simulink model "buck_PV_matematico"  (R2024a)
settings: Solver=FixedStepAuto  StartTime=0.0  StopTime=0.3  FixedStep=1/150000  RelTol=1e-3
values from neighbouring files (symbols this model uses):
  alpha = 0.003177    [parametros.m]
  Cin = 2.7e-3    (= 0.0027)    [parametros.m]
  EG = 1.12    [parametros.m]
  eta = 1.4    [parametros.m]
  Irr = 1.26e-8    (= 1.26e-08)    [parametros.m]
  Isc = 8.21    [parametros.m]
  k = 1.38E-23    (= 1.38e-23)    [parametros.m]
  kdE = 0.1    [parametros.m]
  kE = 0.3333    [parametros.m]
  ki = zeros(n_pontos,n_pontos)    [FLS_dados.m]
  ki_0 = 3.23    [parametros.m]
  kki = 1.5    [parametros.m]
  kkp = 0.0015    [parametros.m]
  kp = zeros(n_pontos,n_pontos)    [FLS_dados.m]
  kp_0 = 0.0055    [parametros.m]
  L = 22.109e-6    (= 2.2109e-05)    [parametros.m]
  n_cell = 45    [parametros.m]
  n_pontos = 21    [FLS_dados.m]
  q = 1.6E-19    (= 1.6e-19)    [parametros.m]
  Rcin = 6.519e-3    (= 0.006519)    [parametros.m]
  Rl = 3e-3    (= 0.003)    [parametros.m]
  Ron = 0.15    [parametros.m]
  Rp_cell = 2.116    [parametros.m]
  Rs_cell = 0.0045    [parametros.m]
  Tr = 298    [parametros.m]
  Vbat = 12    [parametros.m]
  Vto = 1    [parametros.m]
libraries: simulink x1
settings Model: Creator=mario  LastModifiedBy=mario

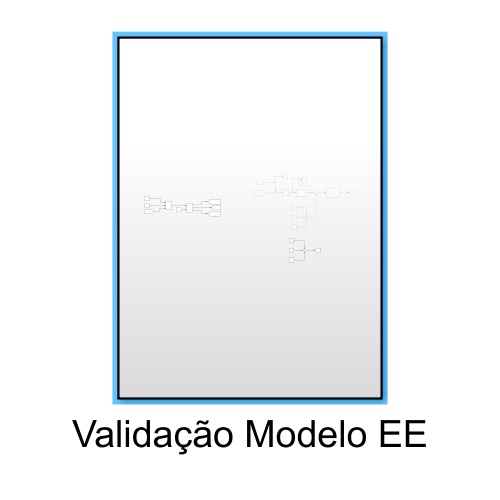
[thumbnail: Simulink's stored preview of the top-level diagram]
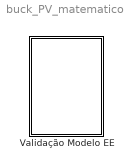
== system buck_PV_matematico ==
  Validação Modelo EE : Subsystem

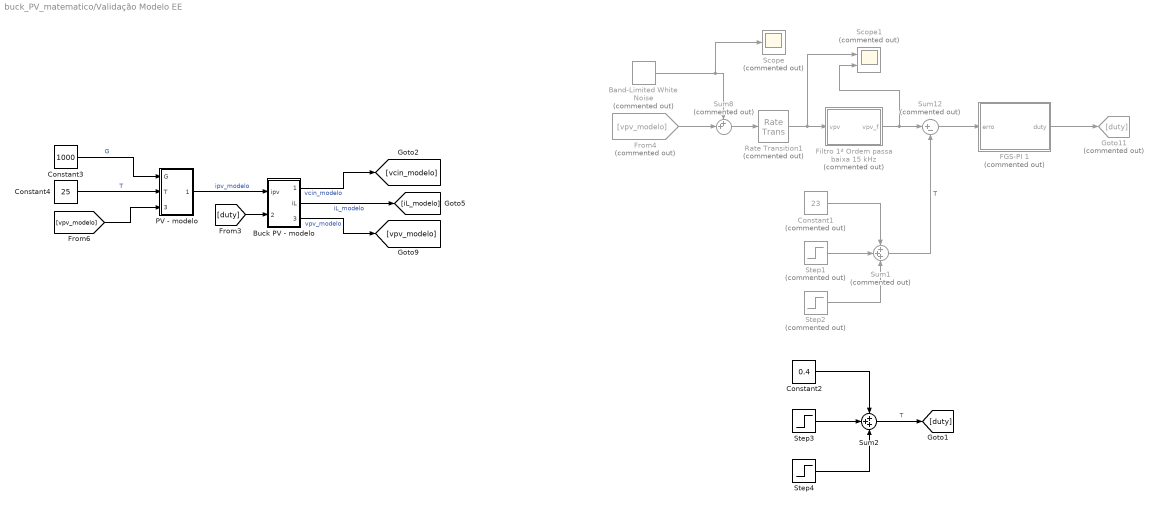
== system buck_PV_matematico/Validação Modelo EE ==
  Band-Limited White Noise : simulink/Sources/Band-Limited White Noise  Commented=on  Cov=[5e-7]  Ts=(1/150000)  seed=[23341]
  Buck PV - modelo : Subsystem
  Constant1 : Constant  Commented=on  Value=23
  Constant2 : Constant  Value=0.4
  Constant3 : Constant  Value=1000
  Constant4 : Constant  Value=25
  FGS-PI 1 : Subsystem  Commented=on
  Filtro 1ª Ordem passa baixa 15 kHz : MATLAB Function  Commented=on  TreatAsAtomicUnit=on
  From4 : From  Commented=on  GotoTag=vpv_modelo
  Goto11 : Goto  Commented=on  GotoTag=duty
  PV - modelo : Subsystem
  Rate Transition1 : RateTransition  Commented=on  OutPortSampleTime=1/150000
  Scope : Scope  Commented=on
  Scope1 : Scope  Commented=on  NumInputPorts=2
  Step1 : Step  Commented=on  Time=0.1  After=3  SampleTime=0
  Step2 : Step  Commented=on  Time=0.2  After=-3  SampleTime=0
  Step3 : Step  Time=0.1  After=0.01  SampleTime=0
  Step4 : Step  Time=0.2  After=-0.01  SampleTime=0
  Sum1 : Sum  Commented=on  Inputs=+++
  Sum12 : Sum  Commented=on  Inputs=|+-
  Sum2 : Sum  Inputs=+++
  Sum8 : Sum  Commented=on  Inputs=++|
  wires:
  PV - modelo/1(Ipv) -> Buck PV - modelo/1(ipv)  "ipv_modelo"
  [duty] -> Buck PV - modelo/2(duty)
  Buck PV - modelo/1(vcin) -> [vcin_modelo]  "vcin_modelo"
  [vpv_modelo] -> PV - modelo/3(Vpv)
  Constant4/1 -> PV - modelo/2(T)  "T"
  Buck PV - modelo/2(iL) -> [iL_modelo]  "iL_modelo"
  Buck PV - modelo/3(vpv) -> [vpv_modelo]  "vpv_modelo"
  Constant3/1 -> PV - modelo/1(G)  "G"
  FGS-PI 1/1(duty) -> Goto11/1
  From4/1 -> Sum8/2
  Band-Limited White Noise/1 -> Scope/1, Sum8/1
  Rate Transition1/1 -> Scope1/1, Filtro 1ª Ordem passa baixa 15 kHz/1(vpv)
  Sum8/1 -> Rate Transition1/1
  Filtro 1ª Ordem passa baixa 15 kHz/1(vpv_f) -> Scope1/2, Sum12/1
  Sum12/1 -> FGS-PI 1/1(erro)
  Step1/1 -> Sum1/2
  Sum1/1 -> Sum12/2  "T"
  Constant1/1 -> Sum1/1
  Step2/1 -> Sum1/3
  Step4/1 -> Sum2/3
  Constant2/1 -> Sum2/1
  Step3/1 -> Sum2/2
  Sum2/1 -> [duty]  "T"

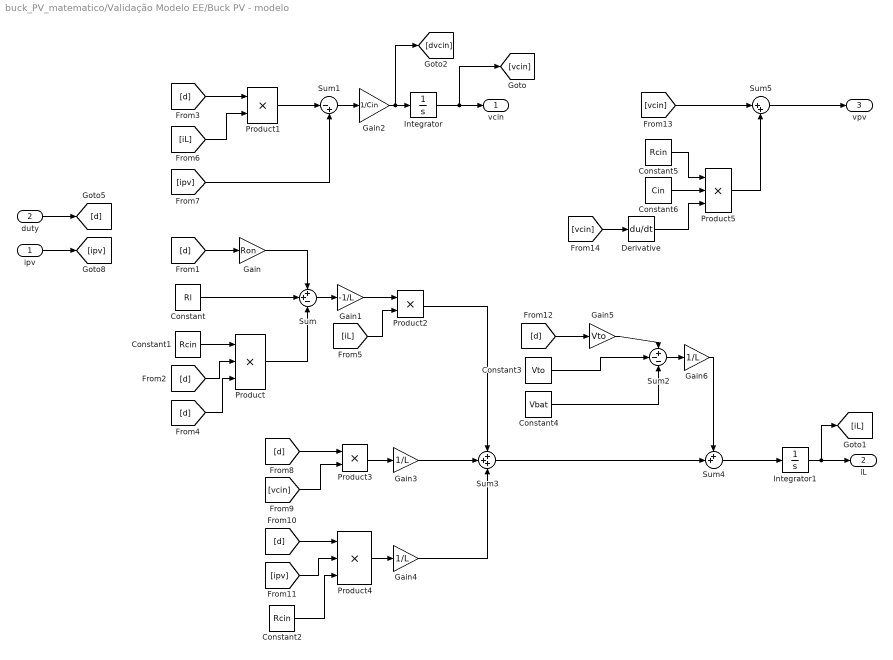
== system buck_PV_matematico/Validação Modelo EE/Buck PV - modelo ==
  ipv : Inport
  duty : Inport  Port=2
  Constant : Constant  Value=Rl
  Constant1 : Constant  Value=Rcin
  Constant2 : Constant  Value=Rcin
  Constant3 : Constant  Value=Vto
  Constant4 : Constant  Value=Vbat
  Constant5 : Constant  Value=Rcin
  Constant6 : Constant  Value=Cin
  Derivative : Derivative
  Gain : Gain  Gain=Ron
  Gain1 : Gain  Gain=-1/L
  Gain2 : Gain  Gain=1/Cin
  Gain3 : Gain  Gain=1/L
  Gain4 : Gain  Gain=1/L
  Gain5 : Gain  Gain=Vto
  Gain6 : Gain  Gain=1/L
  Integrator : Integrator
  Integrator1 : Integrator
  Product : Product  Inputs=3
  Product1 : Product
  Product2 : Product
  Product3 : Product
  Product4 : Product  Inputs=3
  Product5 : Product  Inputs=3
  Sum : Sum  Inputs=++-
  Sum1 : Sum  Inputs=|-+
  Sum2 : Sum  Inputs=+--
  Sum3 : Sum  Inputs=+++
  Sum4 : Sum  Inputs=++|
  Sum5 : Sum  Inputs=|++
  vcin : Outport
  iL : Outport  Port=2
  vpv : Outport  Port=3
  wires:
  ipv/1 -> [ipv]
  duty/1 -> [d]
  Integrator/1 -> [vcin], vcin/1
  Product1/1 -> Sum1/1
  Sum1/1 -> Gain2/1
  [d] -> Product1/1
  [iL] -> Product1/2
  [ipv] -> Sum1/2
  Gain2/1 -> [dvcin], Integrator/1
  [d] -> Gain/1
  Gain/1 -> Sum/1
  Constant/1 -> Sum/2
  Constant1/1 -> Product/1
  [d] -> Product/2
  [d] -> Product/3
  Product/1 -> Sum/3
  Sum/1 -> Gain1/1
  Gain1/1 -> Product2/1
  [iL] -> Product2/2
  [d] -> Product3/1
  [vcin] -> Product3/2
  Product3/1 -> Gain3/1
  [d] -> Product4/1
  [ipv] -> Product4/2
  Constant2/1 -> Product4/3
  Product4/1 -> Gain4/1
  [d] -> Gain5/1
  Gain5/1 -> Sum2/1
  Constant3/1 -> Sum2/2
  Constant4/1 -> Sum2/3
  Gain3/1 -> Sum3/2
  Gain4/1 -> Sum3/3
  Product2/1 -> Sum3/1
  Sum3/1 -> Sum4/2
  Sum2/1 -> Gain6/1
  Sum4/1 -> Integrator1/1
  Integrator1/1 -> [iL], iL/1
  Gain6/1 -> Sum4/1
  [vcin] -> Sum5/1
  Constant6/1 -> Product5/2
  Constant5/1 -> Product5/1
  [vcin] -> Derivative/1
  Product5/1 -> Sum5/2
  Sum5/1 -> vpv/1
  Derivative/1 -> Product5/3

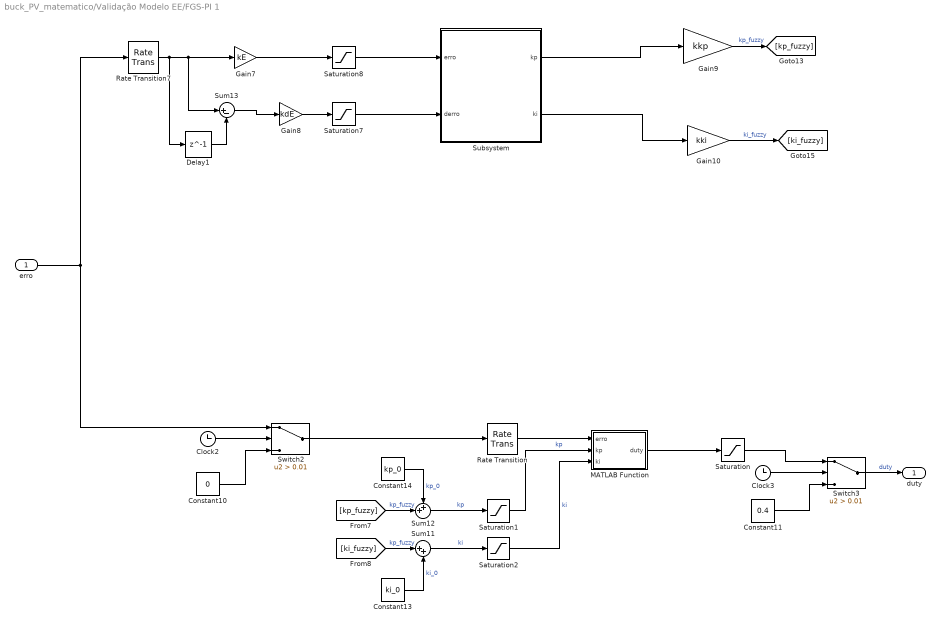
== system buck_PV_matematico/Validação Modelo EE/FGS-PI 1 ==
  erro : Inport
  Clock2 : Clock
  Clock3 : Clock
  Constant10 : Constant  Value=0
  Constant11 : Constant  Value=0.4
  Constant13 : Constant  Value=ki_0
  Constant14 : Constant  Value=kp_0
  Delay1 : Delay  DelayLength=1
  Gain10 : Gain  Gain=kki
  Gain7 : Gain  Gain=kE
  Gain8 : Gain  Gain=kdE
  Gain9 : Gain  Gain=kkp
  MATLAB Function : MATLAB Function  TreatAsAtomicUnit=on
  Rate Transition : RateTransition  OutPortSampleTime=1/150000
  Rate Transition7 : RateTransition  OutPortSampleTime=200e-6
  Saturation : Saturate  UpperLimit=1  LowerLimit=0
  Saturation1 : Saturate  UpperLimit=10  LowerLimit=0
  Saturation2 : Saturate  UpperLimit=10  LowerLimit=0
  Saturation7 : Saturate  UpperLimit=1  LowerLimit=-1
  Saturation8 : Saturate  UpperLimit=1  LowerLimit=-1
  Subsystem : Subsystem
  Sum11 : Sum  Inputs=|++
  Sum12 : Sum  Inputs=++|
  Sum13 : Sum  Inputs=|+-
  Switch2 : Switch  Criteria=u2 > Threshold  Threshold=0.01  SaturateOnIntegerOverflow=off  InputSameDT=off
  Switch3 : Switch  Criteria=u2 > Threshold  Threshold=0.01  SaturateOnIntegerOverflow=off  InputSameDT=off
  duty : Outport
  wires:
  Sum13/1 -> Gain8/1
  Gain7/1 -> Saturation8/1
  Gain9/1 -> [kp_fuzzy]  "kp_fuzzy"
  erro/1 -> Switch2/1, Rate Transition7/1
  Gain8/1 -> Saturation7/1
  Delay1/1 -> Sum13/2
  Constant13/1 -> Sum11/2  "ki_0"
  Gain10/1 -> [ki_fuzzy]  "ki_fuzzy"
  Rate Transition7/1 -> Delay1/1, Sum13/1, Gain7/1
  Rate Transition/1 -> MATLAB Function/1(erro)
  Sum12/1 -> Saturation1/1  "kp"
  Sum11/1 -> Saturation2/1  "ki"
  Constant14/1 -> Sum12/1  "kp_0"
  [kp_fuzzy] -> Sum12/2  "kp_fuzzy"
  [ki_fuzzy] -> Sum11/1  "kp_fuzzy"
  Clock2/1 -> Switch2/2
  Constant10/1 -> Switch2/3
  Switch2/1 -> Rate Transition/1
  Clock3/1 -> Switch3/2
  Constant11/1 -> Switch3/3
  Saturation/1 -> Switch3/1
  Switch3/1 -> duty/1  "duty"
  Saturation1/1 -> MATLAB Function/2(kp)  "kp"
  Saturation2/1 -> MATLAB Function/3(ki)  "ki"
  MATLAB Function/1(duty) -> Saturation/1
  Subsystem/2(ki) -> Gain10/1
  Subsystem/1(kp) -> Gain9/1
  Saturation8/1 -> Subsystem/1(erro)
  Saturation7/1 -> Subsystem/2(derro)

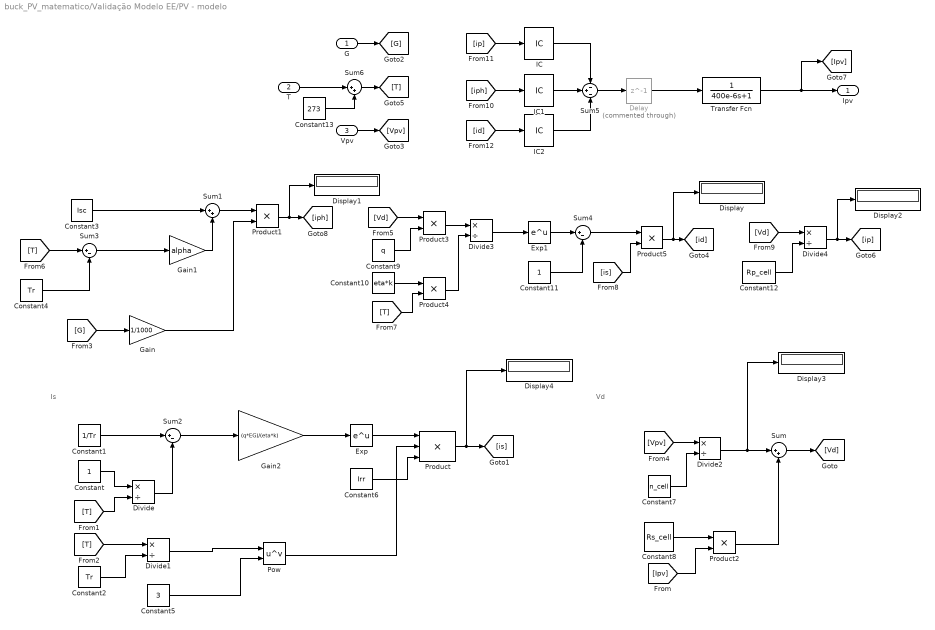
== system buck_PV_matematico/Validação Modelo EE/PV - modelo ==
  note: Vd
  note: Is
  G : Inport
  T : Inport  Port=2
  Vpv : Inport  Port=3
  Constant : Constant
  Constant1 : Constant  Value=1/Tr
  Constant10 : Constant  Value=eta*k
  Constant11 : Constant
  Constant12 : Constant  Value=Rp_cell
  Constant13 : Constant  Value=273
  Constant2 : Constant  Value=Tr
  Constant3 : Constant  Value=Isc
  Constant4 : Constant  Value=Tr
  Constant5 : Constant  Value=3
  Constant6 : Constant  Value=Irr
  Constant7 : Constant  Value=n_cell
  Constant8 : Constant  Value=Rs_cell
  Constant9 : Constant  Value=q
  Delay : Delay  Commented=through  DelayLength=1
  Display{,1..4} (5 alike) : Display
  Divide{,1..4} (5 alike) : Product  Inputs=*/
  Exp : Math
  Exp1 : Math
  Gain : Gain  Gain=1/1000
  Gain1 : Gain  Gain=alpha
  Gain2 : Gain  Gain=(q*EG)/(eta*k)
  IC : InitialCondition  Value=0
  IC1 : InitialCondition  Value=0
  IC2 : InitialCondition  Value=0
  Pow : Math  Operator=pow  SignedPower=on  RndMeth=Zero
  Product : Product  Inputs=3
  Product{1..5} (5 alike) : Product
  Sum : Sum  Inputs=|++
  Sum1 : Sum  Inputs=|++
  Sum2 : Sum  Inputs=|+-
  Sum3 : Sum  Inputs=|+-
  Sum4 : Sum  Inputs=|+-
  Sum5 : Sum  Inputs=-+-
  Sum6 : Sum  Inputs=|++
  Transfer Fcn : TransferFcn  Denominator=[400e-6 1]
  Ipv : Outport
  wires:
  Gain/1 -> Product1/2
  Constant3/1 -> Sum1/1
  G/1 -> [G]
  [G] -> Gain/1
  [T] -> Sum3/1
  Constant4/1 -> Sum3/2
  Sum3/1 -> Gain1/1
  Product1/1 -> Display1/1, [iph]
  Sum1/1 -> Product1/1
  Gain1/1 -> Sum1/2
  [T] -> Divide/2
  Constant/1 -> Divide/1
  Constant1/1 -> Sum2/1
  Divide/1 -> Sum2/2
  Sum2/1 -> Gain2/1
  Gain2/1 -> Exp/1
  Exp/1 -> Product/1
  Constant5/1 -> Pow/2
  Divide1/1 -> Pow/1
  [T] -> Divide1/1
  Constant2/1 -> Divide1/2
  Pow/1 -> Product/2
  Constant6/1 -> Product/3
  Product/1 -> Display4/1, [is]
  Vpv/1 -> [Vpv]
  [Vpv] -> Divide2/1
  Constant7/1 -> Divide2/2
  Divide2/1 -> Display3/1, Sum/1
  Constant8/1 -> Product2/1
  [Ipv] -> Product2/2
  Product2/1 -> Sum/2
  Sum/1 -> [Vd]
  [Vd] -> Product3/1
  Constant9/1 -> Product3/2
  Product3/1 -> Divide3/1
  Constant10/1 -> Product4/1
  [T] -> Product4/2
  Product4/1 -> Divide3/2
  Divide3/1 -> Exp1/1
  Exp1/1 -> Sum4/1
  Constant11/1 -> Sum4/2
  Sum4/1 -> Product5/1
  [is] -> Product5/2
  Product5/1 -> Display/1, [id]
  [Vd] -> Divide4/1
  Constant12/1 -> Divide4/2
  Divide4/1 -> Display2/1, [ip]
  [iph] -> IC1/1
  [ip] -> IC/1
  [id] -> IC2/1
  Sum5/1 -> Delay/1
  Delay/1 -> Transfer Fcn/1
  T/1 -> Sum6/1
  Constant13/1 -> Sum6/2
  Sum6/1 -> [T]
  IC/1 -> Sum5/1
  IC1/1 -> Sum5/2
  IC2/1 -> Sum5/3
  Transfer Fcn/1 -> [Ipv], Ipv/1

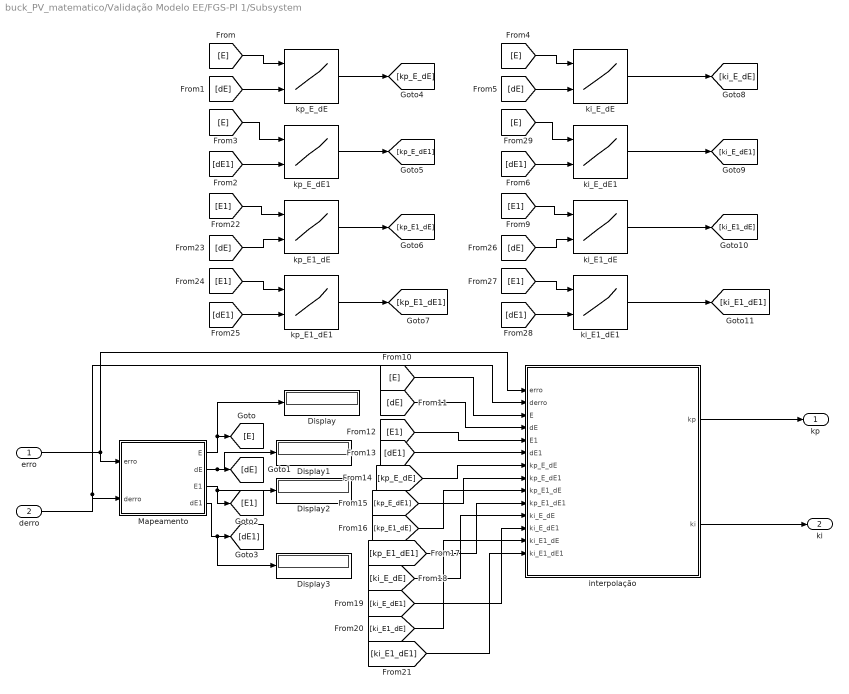
== system buck_PV_matematico/Validação Modelo EE/FGS-PI 1/Subsystem ==
  erro : Inport
  derro : Inport  Port=2
  Display{,1..3} (4 alike) : Display
  Mapeamento : MATLAB Function  TreatAsAtomicUnit=on
  interpolação : MATLAB Function  TreatAsAtomicUnit=on
  ki_E1_dE : Lookup_n-D  LookupTableObject=''  BreakpointsForDimension1=[1:n_pontos]  BreakpointsForDimension2=[1:n_pontos]  BreakpointsForDimension1FirstPoint=10  BreakpointsForDimension2FirstPoint=10  BreakpointsForDimension1Spacing=12  BreakpointsForDimension2Spacing=12  IndexSearchMethod=Evenly spaced points  Table=ki  InterpMethod=Flat  DiagnosticForOutOfRangeInput=Error  InternalRulePriority=Speed  RndMeth=Simplest
      settings: InputPortMap=u0,u1
  ki_E1_dE1 : Lookup_n-D  LookupTableObject=''  BreakpointsForDimension1=[1:n_pontos]  BreakpointsForDimension2=[1:n_pontos]  BreakpointsForDimension1FirstPoint=10  BreakpointsForDimension2FirstPoint=10  BreakpointsForDimension1Spacing=12  BreakpointsForDimension2Spacing=12  IndexSearchMethod=Evenly spaced points  Table=ki  InterpMethod=Flat  DiagnosticForOutOfRangeInput=Error  InternalRulePriority=Speed  RndMeth=Simplest
      settings: InputPortMap=u0,u1
  ki_E_dE : Lookup_n-D  LookupTableObject=''  BreakpointsForDimension1=[1:n_pontos]  BreakpointsForDimension2=[1:n_pontos]  BreakpointsForDimension1FirstPoint=10  BreakpointsForDimension2FirstPoint=10  BreakpointsForDimension1Spacing=12  BreakpointsForDimension2Spacing=12  IndexSearchMethod=Evenly spaced points  Table=ki  InterpMethod=Flat  DiagnosticForOutOfRangeInput=Error  InternalRulePriority=Speed  RndMeth=Simplest
      settings: InputPortMap=u0,u1
  ki_E_dE1 : Lookup_n-D  LookupTableObject=''  BreakpointsForDimension1=[1:n_pontos]  BreakpointsForDimension2=[1:n_pontos]  BreakpointsForDimension1FirstPoint=10  BreakpointsForDimension2FirstPoint=10  BreakpointsForDimension1Spacing=12  BreakpointsForDimension2Spacing=12  IndexSearchMethod=Evenly spaced points  Table=ki  InterpMethod=Flat  DiagnosticForOutOfRangeInput=Error  InternalRulePriority=Speed  RndMeth=Simplest
      settings: InputPortMap=u0,u1
  kp_E1_dE : Lookup_n-D  LookupTableObject=''  BreakpointsForDimension1=[1:n_pontos]  BreakpointsForDimension2=[1:n_pontos]  BreakpointsForDimension1FirstPoint=10  BreakpointsForDimension2FirstPoint=10  BreakpointsForDimension1Spacing=12  BreakpointsForDimension2Spacing=12  IndexSearchMethod=Evenly spaced points  Table=kp  InterpMethod=Flat  DiagnosticForOutOfRangeInput=Error  InternalRulePriority=Speed  RndMeth=Simplest
      settings: InputPortMap=u0,u1
  kp_E1_dE1 : Lookup_n-D  LookupTableObject=''  BreakpointsForDimension1=[1:n_pontos]  BreakpointsForDimension2=[1:n_pontos]  BreakpointsForDimension1FirstPoint=10  BreakpointsForDimension2FirstPoint=10  BreakpointsForDimension1Spacing=12  BreakpointsForDimension2Spacing=12  IndexSearchMethod=Evenly spaced points  Table=kp  InterpMethod=Flat  DiagnosticForOutOfRangeInput=Error  InternalRulePriority=Speed  RndMeth=Simplest
      settings: InputPortMap=u0,u1
  kp_E_dE : Lookup_n-D  LookupTableObject=''  BreakpointsForDimension1=[1:n_pontos]  BreakpointsForDimension2=[1:n_pontos]  BreakpointsForDimension1FirstPoint=10  BreakpointsForDimension2FirstPoint=10  BreakpointsForDimension1Spacing=12  BreakpointsForDimension2Spacing=12  IndexSearchMethod=Evenly spaced points  Table=kp  InterpMethod=Flat  DiagnosticForOutOfRangeInput=Error  InternalRulePriority=Speed  RndMeth=Simplest
      settings: InputPortMap=u0,u1
  kp_E_dE1 : Lookup_n-D  LookupTableObject=''  BreakpointsForDimension1=[1:n_pontos]  BreakpointsForDimension2=[1:n_pontos]  BreakpointsForDimension1FirstPoint=10  BreakpointsForDimension2FirstPoint=10  BreakpointsForDimension1Spacing=12  BreakpointsForDimension2Spacing=12  IndexSearchMethod=Evenly spaced points  Table=kp  InterpMethod=Flat  DiagnosticForOutOfRangeInput=Error  InternalRulePriority=Speed  RndMeth=Simplest
      settings: InputPortMap=u0,u1
  kp : Outport
  ki : Outport  Port=2
  wires:
  [dE] -> interpolação/4(dE)
  [kp_E1_dE1] -> interpolação/10(kp_E1_dE1)
  interpolação/2(ki) -> ki/1
  [E1] -> ki_E1_dE1/1
  [kp_E_dE] -> interpolação/7(kp_E_dE)
  ki_E1_dE1/1 -> [ki_E1_dE1]
  kp_E1_dE/1 -> [kp_E1_dE]
  [E1] -> kp_E1_dE1/1
  [ki_E1_dE] -> interpolação/13(ki_E1_dE)
  [kp_E_dE1] -> interpolação/8(kp_E_dE1)
  [dE] -> kp_E_dE/2
  kp_E1_dE1/1 -> [kp_E1_dE1]
  [E] -> kp_E_dE1/1
  Mapeamento/1(E) -> Display/1, [E]
  derro/1 -> interpolação/2(derro), Mapeamento/2(derro)
  kp_E_dE/1 -> [kp_E_dE]
  [dE1] -> ki_E_dE1/2
  [ki_E_dE] -> interpolação/11(ki_E_dE)
  [ki_E_dE1] -> interpolação/12(ki_E_dE1)
  Mapeamento/4(dE1) -> Display3/1, [dE1]
  Mapeamento/2(dE) -> Display1/1, [dE]
  [E] -> interpolação/3(E)
  [dE] -> ki_E1_dE/2
  kp_E_dE1/1 -> [kp_E_dE1]
  [ki_E1_dE1] -> interpolação/14(ki_E1_dE1)
  [E1] -> ki_E1_dE/1
  [kp_E1_dE] -> interpolação/9(kp_E1_dE)
  [E1] -> interpolação/5(E1)
  [dE1] -> kp_E1_dE1/2
  [dE] -> kp_E1_dE/2
  [E] -> kp_E_dE/1
  [dE1] -> kp_E_dE1/2
  interpolação/1(kp) -> kp/1
  [E] -> ki_E_dE/1
  [E1] -> kp_E1_dE/1
  [dE] -> ki_E_dE/2
  ki_E1_dE/1 -> [ki_E1_dE]
  [E] -> ki_E_dE1/1
  [dE1] -> ki_E1_dE1/2
  ki_E_dE/1 -> [ki_E_dE]
  [dE1] -> interpolação/6(dE1)
  ki_E_dE1/1 -> [ki_E_dE1]
  erro/1 -> Mapeamento/1(erro), interpolação/1(erro)
  Mapeamento/3(E1) -> Display2/1, [E1]

== matlab function buck_PV_matematico/Validação Modelo EE/FGS-PI 1/Subsystem/Mapeamento ==
  data: erro input; E output; derro input; dE output; E1 output; dE1 output
function [E, dE, E1, dE1] = fcn(erro, derro)
   persistent ek_1;
   n_pontos = 21;

    if(isempty(ek_1)) ek_1=0; end

    E = (floor(((n_pontos-1)/2)*erro + ((n_pontos-1)/2)+1));
    dE = (floor(((n_pontos-1)/2)*derro + ((n_pontos-1)/2)+1));
    if(E+1 > n_pontos)
        E1 = E;
    else
        E1 = E+1;
    end

    if(dE+1 > n_pontos)
        dE1 = dE;
    else
        dE1 = dE+1;
    end

== matlab function buck_PV_matematico/Validação Modelo EE/FGS-PI 1/Subsystem/interpolação ==
  data: erro input; kp output; derro input; ki output; E input; dE input; E1 input; dE1 input; kp_E_dE input; kp_E_dE1 input; kp_E1_dE input; kp_E1_dE1 input; ki_E_dE input; ki_E_dE1 input; ki_E1_dE input; ki_E1_dE1 input
function [kp, ki] = fcn(erro, derro, E, dE, E1, dE1, kp_E_dE, kp_E_dE1, kp_E1_dE, kp_E1_dE1, ki_E_dE, ki_E_dE1, ki_E1_dE, ki_E1_dE1)
    
    if (E == E1 || dE == dE1)
        kp = kp_E_dE;
        ki = ki_E_dE;
    else
        n = 21;
        erro_E = (2/(n-1))*(E-1 - ((n-1)/2));
        derro_dE = (2/(n-1))*(dE-1 - ((n-1)/2));
        erro_E1 = (2/(n-1))*(E1-1 - ((n-1)/2));
        derro_dE1 = (2/(n-1))*(dE1-1 - ((n-1)/2));
    
        kp_erro_dE = ((kp_E1_dE - kp_E_dE)/(erro_E1 - erro_E))*(erro-erro_E)+kp_E_dE;
        ki_erro_dE = ((ki_E1_dE - ki_E_dE)/(erro_E1 - erro_E))*(erro-erro_E)+ki_E_dE;
    
        kp_erro_dE1 = ((kp_E1_dE1 - kp_E_dE1)/(erro_E1-erro_E))*(erro-erro_E)+kp_E_dE1;
        ki_erro_dE1 = ((ki_E1_dE1 - ki_E_dE1)/(erro_E1-erro_E))*(erro-erro_E)+ki_E_dE1;
    
        kp = ((kp_erro_dE1 - kp_erro_dE)/(derro_dE1-derro_dE))*(derro-derro_dE) + kp_erro_dE;
        ki = ((ki_erro_dE1 - ki_erro_dE)/(derro_dE1-derro_dE))*(derro-derro_dE) + ki_erro_dE;
    end

== matlab function buck_PV_matematico/Validação Modelo EE/Filtro 1ª Ordem passa baixa 15 kHz ==
  data: vpv input; vpv_f output
function vpv_f = fcn(vpv)

%Valores p/ fc = 15 kHz
% b0 = 0.23905722;
% b1 = 0.23905722;
% a1 = -0.52188555;

%Valores p/ fc = 1.5 kHz
b0 = 0.030459028;
b1 = 0.030459028;
a1 = -0.93908194;

persistent vpv1 vpv_f1

if(isempty(vpv1)) vpv1=0; end
if(isempty(vpv_f1)) vpv_f1=0; end

vpv_f = (b0*vpv)+(b1*vpv1)-(a1*vpv_f1);
vpv1 = vpv;
vpv_f1 = vpv_f;

== matlab function buck_PV_matematico/Validação Modelo EE/FGS-PI 1/MATLAB Function ==
  settings: updateMethod=DISCRETE
  data: erro input; duty output; kp input; ki input
function duty = fcn(erro, kp, ki)

persistent uk_1 ek_1 erro1 erro_f1
if(isempty(uk_1)) uk_1=0; end
if(isempty(ek_1)) ek_1=0; end


ek = erro;

Ts = (1/150e3);
A = kp+(ki*Ts/2);
B = kp - (ki*Ts/2);

u_PI = A*ek - B*ek_1 + uk_1;

ek_1 = ek;
uk_1 = u_PI;

duty = u_PI;
